simulink model "tres_dummy"  (Simulink 8.6)
settings: Solver=VariableStepDiscrete  StartTime=0.0  StopTime=65  RelTol=1e-3
libraries: tres_simulink_blockset x13
settings Model: Creator=matteo  LastModifiedBy=Paolo
settings DebuggingCC: FcnCallInpInsideContextMsg=EnableAllAsWarning
settings GRTTargetCC: CombineOutputUpdateFcns=on  GRTInterface=off
settings ConfigComp: CovSFcnEnable=off

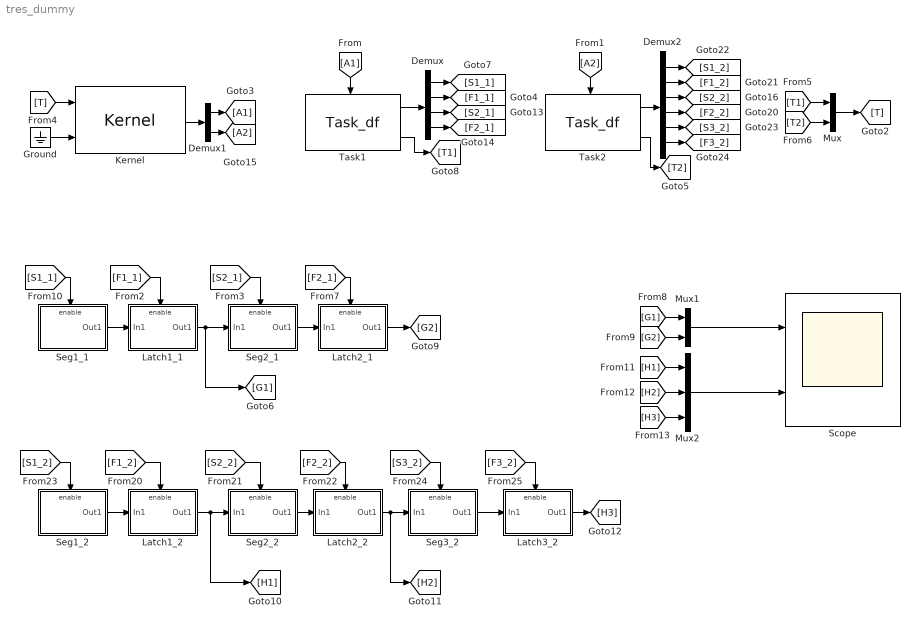
== system tres_dummy ==
  Demux : Demux
  Demux1 : Demux  Outputs=2
  Demux2 : Demux  Outputs=6
  Ground : Ground
  Kernel : tres_simulink_blockset/Kernel  taskset_descr_name=task_set_descr  scheduling_policy=DEADLINE_MONOTONIC  dead_miss_rule=Continue  time_res=Micro_Seconds  core_num=1  under_engine=RTSIM
  Latch1_1 : Subsystem  TreatAsAtomicUnit=on
  Latch1_2 : Subsystem  TreatAsAtomicUnit=on
  Latch2_1 : Subsystem  TreatAsAtomicUnit=on
  Latch2_2 : Subsystem  TreatAsAtomicUnit=on
  Latch3_2 : Subsystem  TreatAsAtomicUnit=on
  Mux : Mux  Inputs=2
  Mux1 : Mux  Inputs=2
  Mux2 : Mux  Inputs=3
  Scope : Scope  NumInputPorts=2
  Seg1_1 : Subsystem  TreatAsAtomicUnit=on
  Seg1_2 : Subsystem  TreatAsAtomicUnit=on
  Seg2_1 : Subsystem  TreatAsAtomicUnit=on
  Seg2_2 : Subsystem  TreatAsAtomicUnit=on
  Seg3_2 : Subsystem  TreatAsAtomicUnit=on
  Task1 : tres_simulink_blockset/Task_df  conf_name=t1_instrs
  Task2 : tres_simulink_blockset/Task_df  conf_name=t2_instrs
  wires:
  [T] -> Kernel/1
  [T1] -> Mux/1
  [T2] -> Mux/2
  Mux/1 -> [T]
  Task2/2 -> [T2]
  Task2/1 -> Demux2/1
  Task1/2 -> [T1]
  Seg1_1/1(Out1) -> Latch1_1/1(In1)
  Latch1_1/1(Out1) -> Seg2_1/1(In1), [G1]
  Seg2_1/1(Out1) -> Latch2_1/1(In1)
  Latch2_1/1(Out1) -> [G2]
  [G1] -> Mux1/1
  [G2] -> Mux1/2
  Mux1/1 -> Scope/1
  Seg1_2/1(Out1) -> Latch1_2/1(In1)
  Seg2_2/1(Out1) -> Latch2_2/1(In1)
  Latch2_2/1(Out1) -> Seg3_2/1(In1), [H2]
  [H1] -> Mux2/1
  [H2] -> Mux2/2
  Latch1_2/1(Out1) -> Seg2_2/1(In1), [H1]
  Seg3_2/1(Out1) -> Latch3_2/1(In1)
  Latch3_2/1(Out1) -> [H3]
  [H3] -> Mux2/3
  Mux2/1 -> Scope/2
  Ground/1 -> Kernel/2
  Task1/1 -> Demux/1
  Demux/1 -> [S1_1]
  Demux/2 -> [F1_1]
  Demux/3 -> [S2_1]
  Demux/4 -> [F2_1]
  Kernel/1 -> Demux1/1
  Demux1/2 -> [A2]
  Demux1/1 -> [A1]
  Demux2/1 -> [S1_2]
  Demux2/2 -> [F1_2]
  Demux2/3 -> [S2_2]
  Demux2/4 -> [F2_2]
  Demux2/5 -> [S3_2]
  Demux2/6 -> [F3_2]
  [A2] -> Task2/Trigger
  [A1] -> Task1/Trigger
  [S1_2] -> Seg1_2/Enable
  [F1_2] -> Latch1_2/Enable
  [S2_2] -> Seg2_2/Enable
  [F2_2] -> Latch2_2/Enable
  [S3_2] -> Seg3_2/Enable
  [F3_2] -> Latch3_2/Enable
  [S1_1] -> Seg1_1/Enable
  [F1_1] -> Latch1_1/Enable
  [S2_1] -> Seg2_1/Enable
  [F2_1] -> Latch2_1/Enable

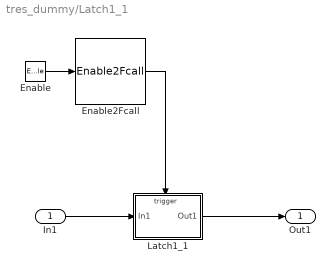
== system tres_dummy/Latch1_1 ==
  In1 : Inport
  Enable : EnablePort  ShowOutputPort=on
  Enable2Fcall : tres_simulink_blockset/Enable2Fcall
  Latch1_1 : Subsystem  TreatAsAtomicUnit=on
  Out1 : Outport
  wires:
  Enable2Fcall/1 -> Latch1_1/Trigger
  Enable/1 -> Enable2Fcall/1
  In1/1 -> Latch1_1/1(In1)
  Latch1_1/1(Out1) -> Out1/1

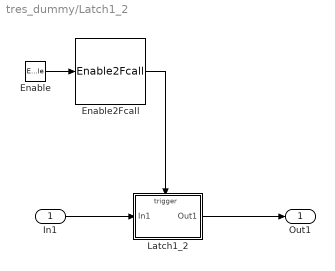
== system tres_dummy/Latch1_2 ==
  In1 : Inport
  Enable : EnablePort  ShowOutputPort=on
  Enable2Fcall : tres_simulink_blockset/Enable2Fcall
  Latch1_2 : Subsystem  TreatAsAtomicUnit=on
  Out1 : Outport
  wires:
  Enable2Fcall/1 -> Latch1_2/Trigger
  Enable/1 -> Enable2Fcall/1
  In1/1 -> Latch1_2/1(In1)
  Latch1_2/1(Out1) -> Out1/1

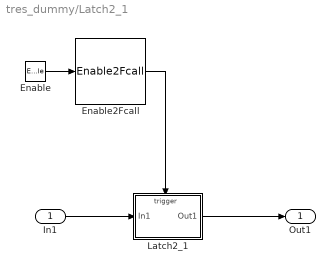
== system tres_dummy/Latch2_1 ==
  In1 : Inport
  Enable : EnablePort  ShowOutputPort=on
  Enable2Fcall : tres_simulink_blockset/Enable2Fcall
  Latch2_1 : Subsystem  TreatAsAtomicUnit=on
  Out1 : Outport
  wires:
  Enable2Fcall/1 -> Latch2_1/Trigger
  Enable/1 -> Enable2Fcall/1
  In1/1 -> Latch2_1/1(In1)
  Latch2_1/1(Out1) -> Out1/1

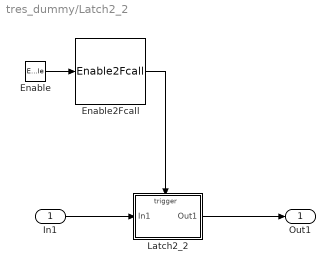
== system tres_dummy/Latch2_2 ==
  In1 : Inport
  Enable : EnablePort  ShowOutputPort=on
  Enable2Fcall : tres_simulink_blockset/Enable2Fcall
  Latch2_2 : Subsystem  TreatAsAtomicUnit=on
  Out1 : Outport
  wires:
  Enable2Fcall/1 -> Latch2_2/Trigger
  Enable/1 -> Enable2Fcall/1
  In1/1 -> Latch2_2/1(In1)
  Latch2_2/1(Out1) -> Out1/1

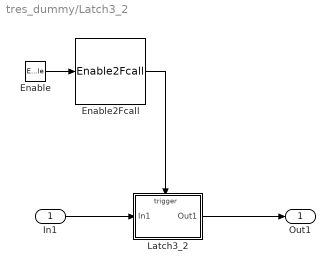
== system tres_dummy/Latch3_2 ==
  In1 : Inport
  Enable : EnablePort  ShowOutputPort=on
  Enable2Fcall : tres_simulink_blockset/Enable2Fcall
  Latch3_2 : Subsystem  TreatAsAtomicUnit=on
  Out1 : Outport
  wires:
  Enable2Fcall/1 -> Latch3_2/Trigger
  Enable/1 -> Enable2Fcall/1
  In1/1 -> Latch3_2/1(In1)
  Latch3_2/1(Out1) -> Out1/1

== system tres_dummy/Seg1_1 ==
  Enable : EnablePort  ShowOutputPort=on
  Enable2Fcall : tres_simulink_blockset/Enable2Fcall
  Seg1_1 : Subsystem  TreatAsAtomicUnit=on
  Out1 : Outport
  wires:
  Enable2Fcall/1 -> Seg1_1/Trigger
  Seg1_1/1(Out1) -> Out1/1
  Enable/1 -> Enable2Fcall/1

== system tres_dummy/Seg1_2 ==
  Enable : EnablePort  ShowOutputPort=on
  Enable2Fcall : tres_simulink_blockset/Enable2Fcall
  Seg1_2 : Subsystem  TreatAsAtomicUnit=on
  Out1 : Outport
  wires:
  Enable2Fcall/1 -> Seg1_2/Trigger
  Seg1_2/1(Out1) -> Out1/1
  Enable/1 -> Enable2Fcall/1

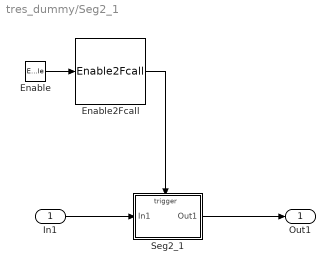
== system tres_dummy/Seg2_1 ==
  In1 : Inport
  Enable : EnablePort  ShowOutputPort=on
  Enable2Fcall : tres_simulink_blockset/Enable2Fcall
  Seg2_1 : Subsystem  TreatAsAtomicUnit=on
  Out1 : Outport
  wires:
  Enable2Fcall/1 -> Seg2_1/Trigger
  Enable/1 -> Enable2Fcall/1
  In1/1 -> Seg2_1/1(In1)
  Seg2_1/1(Out1) -> Out1/1

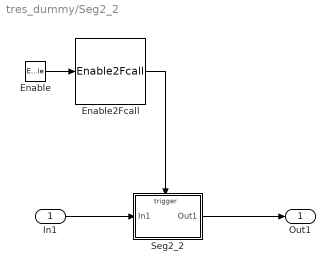
== system tres_dummy/Seg2_2 ==
  In1 : Inport
  Enable : EnablePort  ShowOutputPort=on
  Enable2Fcall : tres_simulink_blockset/Enable2Fcall
  Seg2_2 : Subsystem  TreatAsAtomicUnit=on
  Out1 : Outport
  wires:
  Enable2Fcall/1 -> Seg2_2/Trigger
  Enable/1 -> Enable2Fcall/1
  In1/1 -> Seg2_2/1(In1)
  Seg2_2/1(Out1) -> Out1/1

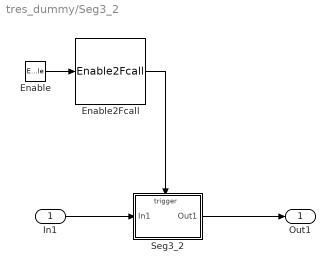
== system tres_dummy/Seg3_2 ==
  In1 : Inport
  Enable : EnablePort  ShowOutputPort=on
  Enable2Fcall : tres_simulink_blockset/Enable2Fcall
  Seg3_2 : Subsystem  TreatAsAtomicUnit=on
  Out1 : Outport
  wires:
  Enable2Fcall/1 -> Seg3_2/Trigger
  Enable/1 -> Enable2Fcall/1
  In1/1 -> Seg3_2/1(In1)
  Seg3_2/1(Out1) -> Out1/1

== system tres_dummy/Latch1_1/Latch1_1 ==
  In1 : Inport
  function : TriggerPort  TriggerType=function-call
  Out1 : Outport
  wires:
  In1/1 -> Out1/1

== system tres_dummy/Latch1_2/Latch1_2 ==
  In1 : Inport
  function : TriggerPort  TriggerType=function-call
  Out1 : Outport
  wires:
  In1/1 -> Out1/1

== system tres_dummy/Latch2_1/Latch2_1 ==
  In1 : Inport
  function : TriggerPort  TriggerType=function-call
  Out1 : Outport
  wires:
  In1/1 -> Out1/1

== system tres_dummy/Latch2_2/Latch2_2 ==
  In1 : Inport
  function : TriggerPort  TriggerType=function-call
  Out1 : Outport
  wires:
  In1/1 -> Out1/1

== system tres_dummy/Latch3_2/Latch3_2 ==
  In1 : Inport
  function : TriggerPort  TriggerType=function-call
  Out1 : Outport
  wires:
  In1/1 -> Out1/1

== system tres_dummy/Seg1_1/Seg1_1 ==
  function : TriggerPort  TriggerType=function-call
  Digital Clock : DigitalClock  SampleTime=-1
  Out1 : Outport
  wires:
  Digital Clock/1 -> Out1/1

== system tres_dummy/Seg1_2/Seg1_2 ==
  function : TriggerPort  TriggerType=function-call
  Digital Clock : DigitalClock  SampleTime=-1
  Out1 : Outport
  wires:
  Digital Clock/1 -> Out1/1

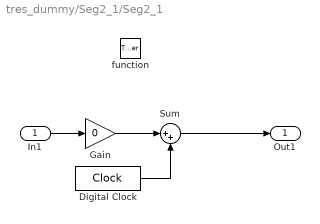
== system tres_dummy/Seg2_1/Seg2_1 ==
  In1 : Inport
  function : TriggerPort  TriggerType=function-call
  Digital Clock : DigitalClock  SampleTime=-1
  Gain : Gain  Gain=0
  Sum : Sum  Inputs=|++
  Out1 : Outport
  wires:
  Sum/1 -> Out1/1
  Digital Clock/1 -> Sum/2
  In1/1 -> Gain/1
  Gain/1 -> Sum/1

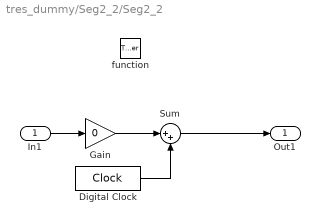
== system tres_dummy/Seg2_2/Seg2_2 ==
  In1 : Inport
  function : TriggerPort  TriggerType=function-call
  Digital Clock : DigitalClock  SampleTime=-1
  Gain : Gain  Gain=0
  Sum : Sum  Inputs=|++
  Out1 : Outport
  wires:
  Sum/1 -> Out1/1
  Digital Clock/1 -> Sum/2
  In1/1 -> Gain/1
  Gain/1 -> Sum/1

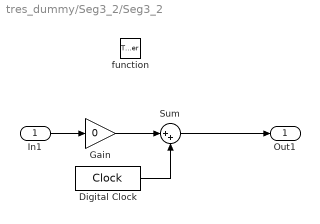
== system tres_dummy/Seg3_2/Seg3_2 ==
  In1 : Inport
  function : TriggerPort  TriggerType=function-call
  Digital Clock : DigitalClock  SampleTime=-1
  Gain : Gain  Gain=0
  Sum : Sum  Inputs=|++
  Out1 : Outport
  wires:
  Sum/1 -> Out1/1
  Digital Clock/1 -> Sum/2
  In1/1 -> Gain/1
  Gain/1 -> Sum/1
